simulink model "digitalIn"  (R2025b)
settings: Solver=ode3  StartTime=0.0  StopTime=Inf  RelTol=1e-3  EnableMultiTasking=on
undefined symbols (not defined in the file): Green, led0
libraries: raspberrypiBasiclib x3, simulink x1
settings Model: FPTRunName=Active  ExtModeTrigDuration=2  Creator=Soochan Kim  LastModifiedBy=Soochan Kim
settings SolverCC: AlgebraicLoopSolver=TrustRegion  PositivePriorityOrder=on
settings DataIOCC: LimitDataPoints=on  SaveFormat=Array
settings OptimizationCC: ExpressionDepthLimit=2147483647.0  LifeSpan=Inf  MaxStackSize=200000
settings DebuggingCC: UnderspecifiedInitializationDetection=Classic  MergeDetectMultiDrivingBlocksExec=none  FcnCallInpInsideContextMsg=warning  UnconnectedInputMsg=warning  UnconnectedOutputMsg=warning  UnconnectedLineMsg=warning  AllowSymbolicDim=off  StateNameClashWarn=warning  SubsystemReferenceDiagnosticForUnitTest=warning  SFUnexpectedBacktrackingDiag=warning  SFNoUnconditionalDefaultTransitionDiag=warning  SFExecutionAtInitializationDiag=none  ArithmeticOperatorsInVariantConditions=warning
settings HardwareCC: ProdBitPerLong=64.0  ProdLargestAtomicInteger=LongLong  ProdLargestAtomicFloat=Double  ProdLongLongMode=on  ProdHWDeviceType=ARM Compatible->ARM Cortex-A (64-bit)
settings ModelReferenceCC: EnableRefExpFcnMdlSchedulingChecks=on  PropagateSignalLabelsOutOfModel=off
settings SFSimCC: SimUseLocalCustomCode=off  CustomCodeUndefinedFunction=UseInterfaceOnly
settings RTWCC: SystemTargetFile=ert.tlc  HardwareBoard=Raspberry Pi (64bit)  TemplateMakefile=ert_default_tmf  RTWVerbose=off  RTWUseLocalCustomCode=off  Toolchain=GNU GCC Embedded Linux  BuildConfiguration=Faster Runs  GPUComputeCapability=3.5  Description=Embedded Coder
settings CodeAppCC: StateflowObjectComments=on
settings ERTTargetCC: ExtModeTransport=2.0  ExtModeStaticAlloc=on  ExtModeMexFile=ext_xcp  ExtModeIntrfLevel=Level2 - Open  InlinedParameterPlacement=Hierarchical  ConvertIfToSwitch=off  SuppressUnreachableDefaultCases=off  DynamicArrayContainerType=coder::array  CodeReplacementLibrary=ARM Cortex-A CMSIS  MultiwordLength=2048.0  ERTCustomFileBanners=off  SupportContinuousTime=on  SupportNonInlinedSFcns=on  RemoveResetFunc=off  SupportVariableSizeSignals=on  ModelStepFunctionPrototypeControlCompliant=off
settings ConfigComp: CovMetricSettings=dw  CovSaveCumulativeToWorkspaceVar=on  CovSaveSingleToWorkspaceVar=on  CovExternalEMLEnable=off  CovSFcnEnable=off

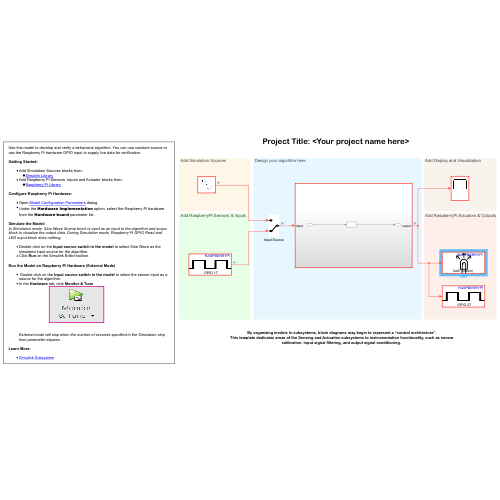
[thumbnail: Simulink's stored preview of the top-level diagram]
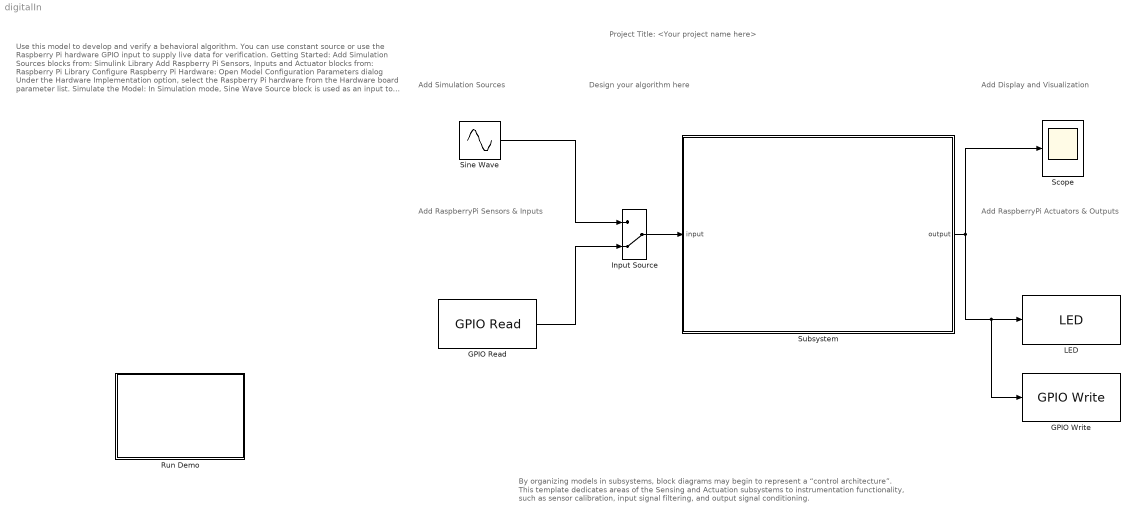
== system digitalIn ==
  note: Use this model to develop and verify a behavioral algorithm. You can use constant source or use the Raspberry Pi hardware GPIO input to supply live data for verification.
      |
      | Getting Started:
      |
      | Add Simulation Sources blocks from:
      | Simulink Library
      | Add Raspberry Pi Sensors, Inputs and Actuator blocks from:
      | Raspberry Pi Library
      |
      | Configure Raspberry Pi Hardware:
      |
      | Open Model Configuration Parameters dialog
      | Under the Hardware Implementation option, select the Raspberry Pi hardware from the Hardware board parameter list.
      |
      | Simulate the Model:
      | In Simulation mode, Sine Wave Source block is used as an input to the algorithm and scope block to visualize the output data. During Simulation mode, Raspberry Pi GPIO Read and LED ouput block does nothing.
      |
      | Double click on the Input source switch in the model to select Sine Wave as the simulated input source for the algorithm.
      | Click Run on the Simulink Editor toolbar.
      |
      | Run the Model on Raspberry Pi Hardware (External Mode)
      |
      | Double click on the Input source switch in the model to select the sensor input as a source for the algorithm.
      | In the Hardware tab, click Monitor & Tune
      |
      | External mode will stop when the number of seconds specified in the Simulation stop time parameter elapses.
      |
      | Learn More:
      |
      | Simulink Subsystem
  note: By organizing models in subsystems, block diagrams may begin to represent a “control architecture”.
      | This template dedicates areas of the Sensing and Actuation subsystems to instrumentation functionality, such as sensor calibration, input signal filtering, and output signal conditioning.
  note: Add Display and Visualization
  note: Add RaspberryPi Actuators & Outputs
  note: Add Simulation Sources
  note: Project Title: <Your project name here>
  note: Design your algorithm here
  note: Add RaspberryPi Sensors & Inputs
  GPIO Read : raspberrypiBasiclib/GPIO Read  BoardProperty=Pi 4 Model B  gpio=17  SampleTime=-1  blockPlatform=RASPBERRYPI  PinNumber=4  board=[]  direction=[]  internalResistor=[]
  GPIO Write : raspberrypiBasiclib/GPIO Write  BoardProperty=Pi 4 Model B  gpio=27  blockPlatform=Raspberry Pi  PinNumber=17  board=[]  direction=[]
  Input Source : ManualSwitch  CurrentSetting=0
  LED : raspberrypiBasiclib/LED  BoardProperty=Pi 4 Model B  LED_=led0 (Green)
  Run Demo : Subsystem  Description=Controls host-side RTDX processing.
      mask Display: pic=imread('raspberrypiMonitorAndTune.png');image(pic);
  Scope : Scope
      settings: DataLoggingSaveFormat=Array
  Sine Wave : Sin  SineType=Sample based  Amplitude=1000  SampleTime=0.1
  Subsystem : Subsystem
  wires:
  Subsystem/1(output) -> GPIO Write/1, LED/1, Scope/1
  Sine Wave/1 -> Input Source/1
  Input Source/1 -> Subsystem/1(input)
  GPIO Read/1 -> Input Source/2

== system digitalIn/Run Demo ==

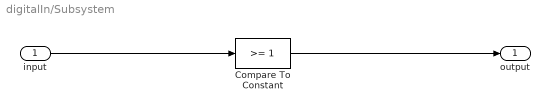
== system digitalIn/Subsystem ==
  input : Inport
  Compare To Constant : simulink/Logic and Bit Operations/Compare To Constant  relop=>=  const=1  OutDataTypeStr=boolean
  output : Outport
  wires:
  Compare To Constant/1 -> output/1
  input/1 -> Compare To Constant/1
